simulink model "user_cmd"  (R2021a)
settings: Solver=FixedStepAuto  StartTime=0.0  StopTime=10.0  RelTol=1e-3
libraries: slrealtimeiplib x9, slrealtimeutilitieslib x7, simulink x5
settings Model: Creator=Ruixuan  LastModifiedBy=icl-baby
settings SolverCC: ConcurrentTasks=on  PositivePriorityOrder=on  AutoInsertRateTranBlk=on  InsertRTBMode=Never (minimum delay)
settings OptimizationCC: BlockReduction=off  DefaultParameterBehavior=Inlined  OptimizeBlockIOStorage=off
settings DebuggingCC: TasksWithSamePriorityMsg=none
settings HardwareCC: ProdBitPerLong=64  ProdLongLongMode=on  ProdHWDeviceType=Intel->x86-64 (Linux 64)
settings ModelReferenceCC: ModelReferenceNumInstancesAllowed=Single
settings RTWCC: Description=Simulink Real-Time  SystemTargetFile=slrealtime.tlc  TemplateMakefile=slrealtime_default_tmf  Toolchain=Simulink Real-Time Toolchain  BuildConfiguration=Faster Runs  CodeExecutionProfiling=on  TargetLang=C++

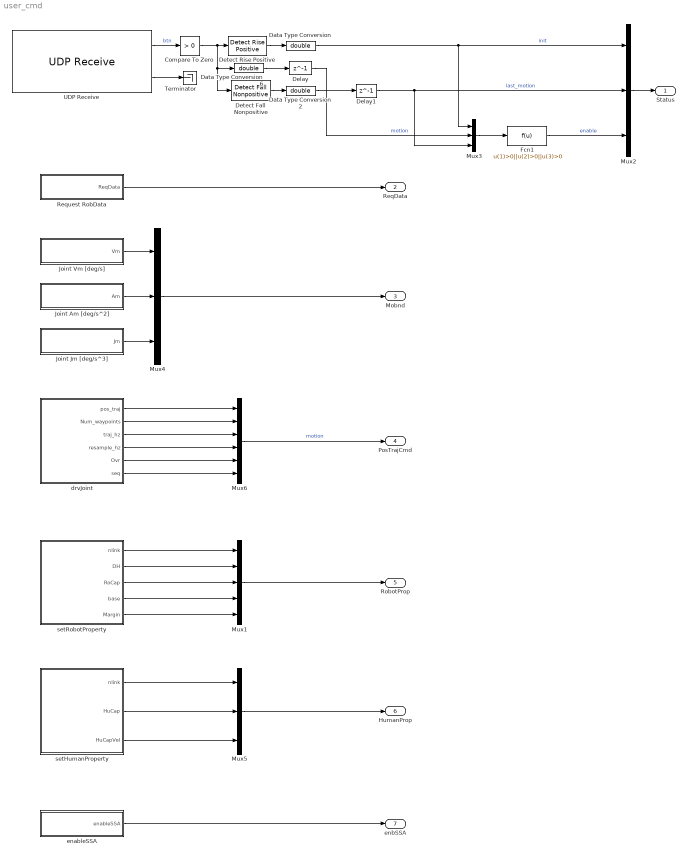
== system user_cmd ==
  Compare To Zero : simulink/Logic and Bit Operations/Compare To Zero  relop=>  OutDataTypeStr=boolean
  Data Type Conversion : DataTypeConversion  OutDataTypeStr=double
  Data Type Conversion2 : DataTypeConversion  OutDataTypeStr=double
  Data Type Conversion6 : DataTypeConversion  OutDataTypeStr=double
  Delay : Delay  DelayLength=1  InitialCondition=0
  Delay1 : Delay  DelayLength=1  InitialCondition=0
  Detect Fall Nonpositive : simulink/Logic and Bit Operations/Detect Fall Nonpositive  vinit=1  OutDataTypeStr=boolean
      settings: SourceProductBaseCode=SL
  Detect Rise Positive : simulink/Logic and Bit Operations/Detect Rise Positive  vinit=0  OutDataTypeStr=boolean
  Fcn1 : Fcn  Expr=u(1)>0||u(2)>0||u(3)>0
  Joint Am [deg/s^2] : Subsystem  mask(CartPosTrjLimit){}
  Joint Jm [deg/s^3] : Subsystem  mask(CartPosTrjLimit){}
  Joint Vm [deg/s] : Subsystem  mask(CartPosTrjLimit){}
  Mux1 : Mux  Inputs=[1,40,70,3,1]
  Mux2 : Mux  Inputs=3
  Mux3 : Mux  Inputs=3
  Mux4 : Mux  Inputs=3
  Mux5 : Mux  Inputs=[1,70,60]
  Mux6 : Mux  Inputs=[11250,1,1,1,1,1]
  Request RobData : Subsystem  mask(CartPosTrjLimit){}
  Terminator : Terminator
  UDP Receive : slrealtimeiplib/UDP Receive  useHostTargetConn=on  ipAddress=10.10.10.15  localPort=8001  rcvWidth=1  rcvFmAny=on  fmAddress=192.168.7.2  sampleTime=Ts
      settings: SourceProductBaseCode=XP
  drvJoint : Subsystem  mask(DesiredPoseUserInput){}
  enableSSA : Subsystem  mask(CartPosTrjLimit){}
  setHumanProperty : Subsystem  mask(DesiredPoseUserInput){}
  setRobotProperty : Subsystem  mask(DesiredPoseUserInput){}
  Status : Outport  VectorParamsAs1DForOutWhenUnconnected=off
  ReqData : Outport  Port=2  VectorParamsAs1DForOutWhenUnconnected=off
  Mobnd : Outport  Port=3  VectorParamsAs1DForOutWhenUnconnected=off
  PosTrajCmd : Outport  Port=4  VectorParamsAs1DForOutWhenUnconnected=off
  RobotProp : Outport  Port=5  VectorParamsAs1DForOutWhenUnconnected=off
  HumanProp : Outport  Port=6  VectorParamsAs1DForOutWhenUnconnected=off
  enbSSA : Outport  Port=7  VectorParamsAs1DForOutWhenUnconnected=off
  wires:
  Compare To Zero/1 -> Detect Fall Nonpositive/1, Data Type Conversion6/1, Detect Rise Positive/1
  Fcn1/1 -> Mux2/3  "enable"
  Mux2/1 -> Status/1
  Data Type Conversion2/1 -> Delay1/1
  Detect Rise Positive/1 -> Data Type Conversion/1
  Delay/1 -> Mux3/2  "motion"
  Detect Fall Nonpositive/1 -> Data Type Conversion2/1
  UDP Receive/2 -> Terminator/1
  Joint Vm [deg/s]/1(Vm) -> Mux4/1
  UDP Receive/1 -> Compare To Zero/1  "btn"
  Mux3/1 -> Fcn1/1
  Delay1/1 -> Mux3/3, Mux2/2  "last_motion"
  drvJoint/3(traj_hz) -> Mux6/3
  Joint Am [deg/s^2]/1(Am) -> Mux4/2
  Data Type Conversion/1 -> Mux3/1, Mux2/1  "init"
  drvJoint/2(Num_waypoints) -> Mux6/2
  Data Type Conversion6/1 -> Delay/1
  drvJoint/1(pos_traj) -> Mux6/1
  Joint Jm [deg/s^3]/1(Jm) -> Mux4/3
  Mux4/1 -> Mobnd/1
  Request RobData/1(ReqData) -> ReqData/1
  drvJoint/6(seq) -> Mux6/6
  drvJoint/5(Ovr) -> Mux6/5
  drvJoint/4(resample_hz) -> Mux6/4
  Mux6/1 -> PosTrajCmd/1  "motion"
  Mux1/1 -> RobotProp/1
  setRobotProperty/5(Margin) -> Mux1/5
  setRobotProperty/4(base) -> Mux1/4
  setRobotProperty/3(RoCap) -> Mux1/3
  setRobotProperty/2(DH) -> Mux1/2
  setRobotProperty/1(nlink) -> Mux1/1
  setHumanProperty/1(nlink) -> Mux5/1
  setHumanProperty/2(HuCap) -> Mux5/2
  Mux5/1 -> HumanProp/1
  enableSSA/1(enableSSA) -> enbSSA/1
  setHumanProperty/3(HuCapVel) -> Mux5/3

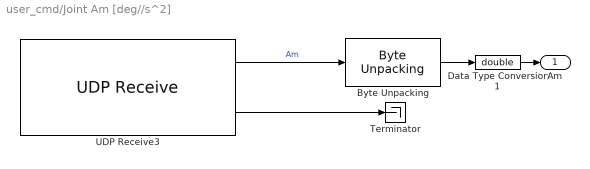
== system user_cmd/Joint Am [deg//s^2] ==
  "Byte Unpacking " : slrealtimeutilitieslib/Byte Unpacking  MaskUnpackedDataTypes={'single'}  MaskUnpackedDataSizes={[6]}  MaskAlignment=1
      settings: SourceProductBaseCode=XP
  Data Type Conversion1 : DataTypeConversion  OutDataTypeStr=double
  Terminator : Terminator
  UDP Receive3 : slrealtimeiplib/UDP Receive  useHostTargetConn=on  ipAddress=10.10.10.15  localPort=8004  rcvWidth=24  rcvFmAny=on  fmAddress=192.168.7.2  sampleTime=Ts
      settings: SourceProductBaseCode=XP
  Am : Outport  VectorParamsAs1DForOutWhenUnconnected=off
  wires:
  UDP Receive3/2 -> Terminator/1
  UDP Receive3/1 -> "Byte Unpacking "/1  "Am"
  "Byte Unpacking "/1 -> Data Type Conversion1/1
  Data Type Conversion1/1 -> Am/1

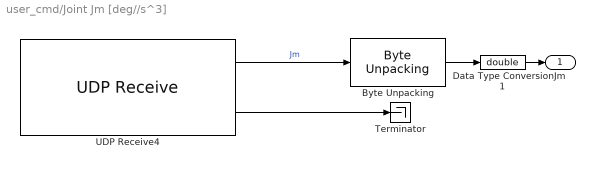
== system user_cmd/Joint Jm [deg//s^3] ==
  "Byte Unpacking " : slrealtimeutilitieslib/Byte Unpacking  MaskUnpackedDataTypes={'single'}  MaskUnpackedDataSizes={[6]}  MaskAlignment=1
      settings: SourceProductBaseCode=XP
  Data Type Conversion1 : DataTypeConversion  OutDataTypeStr=double
  Terminator : Terminator
  UDP Receive4 : slrealtimeiplib/UDP Receive  useHostTargetConn=on  ipAddress=10.10.10.15  localPort=8005  rcvWidth=24  rcvFmAny=on  fmAddress=192.168.7.2  sampleTime=Ts
      settings: SourceProductBaseCode=XP
  Jm : Outport  VectorParamsAs1DForOutWhenUnconnected=off
  wires:
  UDP Receive4/2 -> Terminator/1
  UDP Receive4/1 -> "Byte Unpacking "/1  "Jm"
  "Byte Unpacking "/1 -> Data Type Conversion1/1
  Data Type Conversion1/1 -> Jm/1

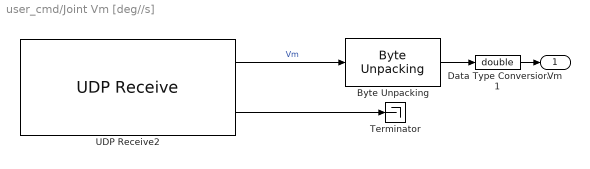
== system user_cmd/Joint Vm [deg//s] ==
  "Byte Unpacking " : slrealtimeutilitieslib/Byte Unpacking  MaskUnpackedDataTypes={'single'}  MaskUnpackedDataSizes={[6]}  MaskAlignment=1
      settings: SourceProductBaseCode=XP
  Data Type Conversion1 : DataTypeConversion  OutDataTypeStr=double
  Terminator : Terminator
  UDP Receive2 : slrealtimeiplib/UDP Receive  useHostTargetConn=on  ipAddress=10.10.10.15  localPort=8003  rcvWidth=24  rcvFmAny=on  fmAddress=192.168.7.2  sampleTime=Ts
      settings: SourceProductBaseCode=XP
  Vm : Outport  VectorParamsAs1DForOutWhenUnconnected=off
  wires:
  UDP Receive2/2 -> Terminator/1
  UDP Receive2/1 -> "Byte Unpacking "/1  "Vm"
  "Byte Unpacking "/1 -> Data Type Conversion1/1
  Data Type Conversion1/1 -> Vm/1

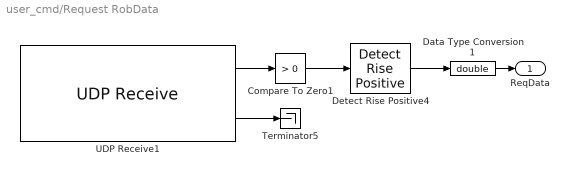
== system user_cmd/Request RobData ==
  Compare To Zero1 : simulink/Logic and Bit Operations/Compare To Zero  relop=>  OutDataTypeStr=boolean
  Data Type Conversion1 : DataTypeConversion  OutDataTypeStr=double
  Detect Rise Positive4 : simulink/Logic and Bit Operations/Detect Rise Positive  vinit=0  OutDataTypeStr=boolean
  Terminator5 : Terminator
  UDP Receive1 : slrealtimeiplib/UDP Receive  useHostTargetConn=on  ipAddress=10.10.10.15  localPort=8106  rcvWidth=1  rcvFmAny=on  fmAddress=0.0.0.0  sampleTime=Ts
      settings: SourceProductBaseCode=XP
  ReqData : Outport  VectorParamsAs1DForOutWhenUnconnected=off
  wires:
  Data Type Conversion1/1 -> ReqData/1
  UDP Receive1/2 -> Terminator5/1
  Compare To Zero1/1 -> Detect Rise Positive4/1
  UDP Receive1/1 -> Compare To Zero1/1
  Detect Rise Positive4/1 -> Data Type Conversion1/1

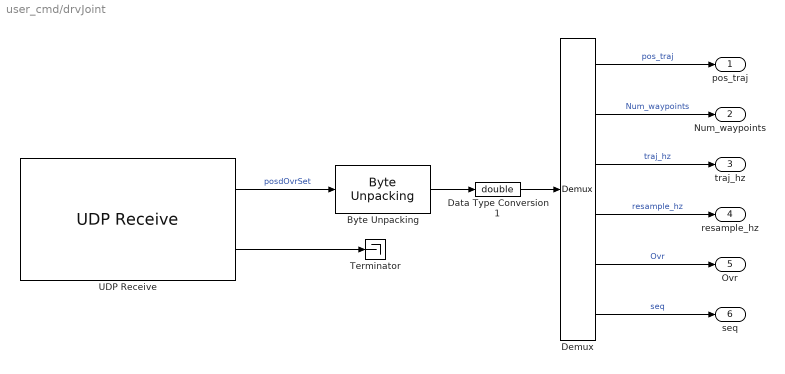
== system user_cmd/drvJoint ==
  "Byte Unpacking " : slrealtimeutilitieslib/Byte Unpacking  MaskUnpackedDataTypes={'single'}  MaskUnpackedDataSizes={[11255]}  MaskAlignment=1
      settings: SourceProductBaseCode=XP
  Data Type Conversion1 : DataTypeConversion  OutDataTypeStr=double
  Demux : Demux  Outputs=[11250,1,1,1,1,1]
      settings: DisplayOption=none
  Terminator : Terminator
  UDP Receive : slrealtimeiplib/UDP Receive  useHostTargetConn=on  ipAddress=10.10.10.15  localPort=8104  rcvWidth=45020  rcvFmAny=on  fmAddress=192.168.7.2  sampleTime=Ts
      settings: SourceProductBaseCode=XP
  pos_traj : Outport  VectorParamsAs1DForOutWhenUnconnected=off
  Num_waypoints : Outport  Port=2  VectorParamsAs1DForOutWhenUnconnected=off
  traj_hz : Outport  Port=3  VectorParamsAs1DForOutWhenUnconnected=off
  resample_hz : Outport  Port=4  VectorParamsAs1DForOutWhenUnconnected=off
  Ovr : Outport  Port=5  VectorParamsAs1DForOutWhenUnconnected=off
  seq : Outport  Port=6  VectorParamsAs1DForOutWhenUnconnected=off
  wires:
  UDP Receive/1 -> "Byte Unpacking "/1  "posdOvrSet"
  "Byte Unpacking "/1 -> Data Type Conversion1/1
  UDP Receive/2 -> Terminator/1
  Data Type Conversion1/1 -> Demux/1
  Demux/1 -> pos_traj/1  "pos_traj"
  Demux/5 -> Ovr/1  "Ovr"
  Demux/6 -> seq/1  "seq"
  Demux/2 -> Num_waypoints/1  "Num_waypoints"
  Demux/3 -> traj_hz/1  "traj_hz"
  Demux/4 -> resample_hz/1  "resample_hz"

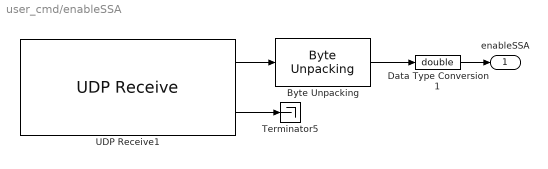
== system user_cmd/enableSSA ==
  "Byte Unpacking " : slrealtimeutilitieslib/Byte Unpacking  MaskUnpackedDataTypes={'single'}  MaskUnpackedDataSizes={[1]}  MaskAlignment=1
      settings: SourceProductBaseCode=XP
  Data Type Conversion1 : DataTypeConversion  OutDataTypeStr=double
  Terminator5 : Terminator
  UDP Receive1 : slrealtimeiplib/UDP Receive  useHostTargetConn=on  ipAddress=10.10.10.15  localPort=8105  rcvWidth=4  rcvFmAny=on  fmAddress=0.0.0.0  sampleTime=Ts
      settings: SourceProductBaseCode=XP
  enableSSA : Outport  VectorParamsAs1DForOutWhenUnconnected=off
  wires:
  Data Type Conversion1/1 -> enableSSA/1
  UDP Receive1/2 -> Terminator5/1
  UDP Receive1/1 -> "Byte Unpacking "/1
  "Byte Unpacking "/1 -> Data Type Conversion1/1

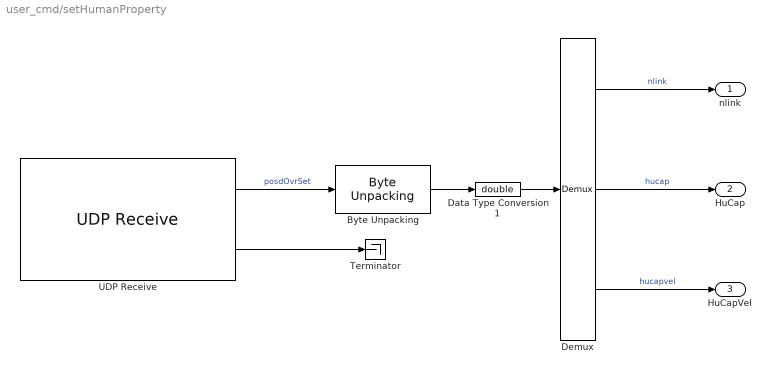
== system user_cmd/setHumanProperty ==
  "Byte Unpacking " : slrealtimeutilitieslib/Byte Unpacking  MaskUnpackedDataTypes={'single'}  MaskUnpackedDataSizes={[131]}  MaskAlignment=1
      settings: SourceProductBaseCode=XP
  Data Type Conversion1 : DataTypeConversion  OutDataTypeStr=double
  Demux : Demux  Outputs=[1,70,60]
      settings: DisplayOption=none
  Terminator : Terminator
  UDP Receive : slrealtimeiplib/UDP Receive  useHostTargetConn=on  ipAddress=10.10.10.15  localPort=8108  rcvWidth=524  rcvFmAny=on  fmAddress=192.168.7.2  sampleTime=Ts
      settings: SourceProductBaseCode=XP
  nlink : Outport  VectorParamsAs1DForOutWhenUnconnected=off
  HuCap : Outport  Port=2  VectorParamsAs1DForOutWhenUnconnected=off
  HuCapVel : Outport  Port=3  VectorParamsAs1DForOutWhenUnconnected=off
  wires:
  UDP Receive/1 -> "Byte Unpacking "/1  "posdOvrSet"
  "Byte Unpacking "/1 -> Data Type Conversion1/1
  UDP Receive/2 -> Terminator/1
  Data Type Conversion1/1 -> Demux/1
  Demux/1 -> nlink/1  "nlink"
  Demux/2 -> HuCap/1  "hucap"
  Demux/3 -> HuCapVel/1  "hucapvel"

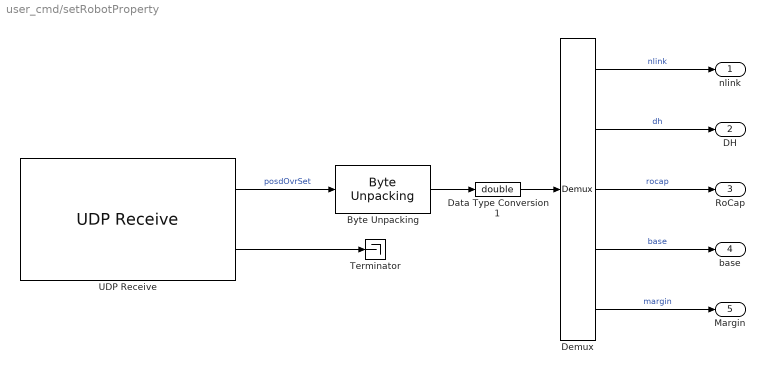
== system user_cmd/setRobotProperty ==
  "Byte Unpacking " : slrealtimeutilitieslib/Byte Unpacking  MaskUnpackedDataTypes={'single'}  MaskUnpackedDataSizes={[115]}  MaskAlignment=1
      settings: SourceProductBaseCode=XP
  Data Type Conversion1 : DataTypeConversion  OutDataTypeStr=double
  Demux : Demux  Outputs=[1,40,70,3,1]
      settings: DisplayOption=none
  Terminator : Terminator
  UDP Receive : slrealtimeiplib/UDP Receive  useHostTargetConn=on  ipAddress=10.10.10.15  localPort=8107  rcvWidth=460  rcvFmAny=on  fmAddress=192.168.7.2  sampleTime=Ts
      settings: SourceProductBaseCode=XP
  nlink : Outport  VectorParamsAs1DForOutWhenUnconnected=off
  DH : Outport  Port=2  VectorParamsAs1DForOutWhenUnconnected=off
  RoCap : Outport  Port=3  VectorParamsAs1DForOutWhenUnconnected=off
  base : Outport  Port=4  VectorParamsAs1DForOutWhenUnconnected=off
  Margin : Outport  Port=5  VectorParamsAs1DForOutWhenUnconnected=off
  wires:
  UDP Receive/1 -> "Byte Unpacking "/1  "posdOvrSet"
  "Byte Unpacking "/1 -> Data Type Conversion1/1
  UDP Receive/2 -> Terminator/1
  Data Type Conversion1/1 -> Demux/1
  Demux/1 -> nlink/1  "nlink"
  Demux/5 -> Margin/1  "margin"
  Demux/2 -> DH/1  "dh"
  Demux/3 -> RoCap/1  "rocap"
  Demux/4 -> base/1  "base"
